simulink model "FrictionID_ref"  (R2022b)
settings: Solver=FixedStepDiscrete  StartTime=0.0  StopTime=160  FixedStep=0.000005  RelTol=1e-3  EnableMultiTasking=on
settings Model: RequirementInfo={} %GIDa_fe9045fd_0412_4b6e_8206_617cc20e6fde  FPTRunName=Active  Creator=ts  LastModifiedBy=hufnagelde
settings SolverCC: AlgebraicLoopSolver=TrustRegion  PositivePriorityOrder=on  AutoInsertRateTranBlk=on
settings DataIOCC: SaveOutput=off  SignalLogging=off  DSMLogging=off  SaveTime=off
settings OptimizationCC: DefaultParameterBehavior=Inlined  UseDivisionForNetSlopeComputation=on  GainParamInheritBuiltInType=on  UseFloatMulNetSlope=on  DefaultUnderspecifiedDataType=single  UseSpecifiedMinMax=on  InlineInvariantSignals=on  PassReuseOutputArgsAs=Individual arguments  ZeroExternalMemoryAtStartup=off  ZeroInternalMemoryAtStartup=off  NoFixptDivByZeroProtection=on  EfficientFloat2IntCast=on  LifeSpan=1  MaxStackSize=64  OptimizeBlockOrder=speed  DifferentSizesBufferReuse=on  EfficientTunableParamExpr=on
settings DebuggingCC: UnconnectedInputMsg=warning  UnconnectedOutputMsg=warning  UnconnectedLineMsg=warning  BusObjectLabelMismatch=error  AllowSymbolicDim=off  SFUnexpectedBacktrackingDiag=warning  SFNoUnconditionalDefaultTransitionDiag=warning  SFExecutionAtInitializationDiag=none  SFMachineParentedDataDiag=warning  ArithmeticOperatorsInVariantConditions=warning
settings HardwareCC: ProdBitPerPointer=32  ProdBitPerSizeT=32  ProdBitPerPtrDiffT=32  ProdLargestAtomicInteger=Long  ProdLargestAtomicFloat=Double  ProdWordSize=32  ProdLongLongMode=on  ProdHWDeviceType=ARM Compatible->ARM Cortex-R  HardwareBoardFeatureSet=SoCBlockset
settings ModelReferenceCC: EnableRefExpFcnMdlSchedulingChecks=on
settings SFSimCC: SimGenImportedTypeDefs=on  MATLABDynamicMemAlloc=off
settings RTWCC: Description=Embedded Coder  SystemTargetFile=ert.tlc  GenCodeOnly=on  TemplateMakefile=ert_default_tmf  GenerateReport=on  BuildConfiguration=Faster Runs  IncludeHyperlinkInReport=on  LaunchReport=on  GenerateTraceInfo=on  GenerateTraceReport=on  GenerateTraceReportSl=on  GenerateTraceReportSf=on  GenerateTraceReportEml=on  GenerateCodeMetricsReport=on  CheckMdlBeforeBuild=Warning  DLArmComputeVersion=19.05
settings CodeAppCC: ForceParamTrailComments=on  IgnoreCustomStorageClasses=off  OperatorAnnotations=on  SimulinkDataObjDesc=on  SFDataObjDesc=on  MATLABFcnDesc=on  CustomSymbolStrGlobalVar=rt$M$R$N  CustomSymbolStrType=$N$M$R_t  CustomSymbolStrFcn=$N$M$F  CustomSymbolStrMacro=$N$M  InsertBlockDesc=on  StateflowObjectComments=on  MATLABSourceComments=on  EnableCustomComments=on  ReqsInCode=on
settings ERTTargetCC: TargetLangStandard=C99 (ISO)  CodeReplacementLibrary=GNU C99 extensions  MultiwordLength=2048  IncludeMdlTerminateFcn=off  CombineSignalStateStructs=on  SuppressErrorStatus=on  IncludeFileDelimiter=UseQuote  SupportAbsoluteTime=off  CodeInterfacePackaging=Reusable function  SupportNonFinite=off  RemoveResetFunc=off  InlinedParameterPlacement=NonHierarchical  MultiInstanceErrorCode=Warning  RootIOFormat=Part of model data structure  ERTCustomFileTemplate=example_file_process.tlc  GlobalDataDefinition=InSourceFile  GlobalDataReference=InSourceFile  ERTFilePackagingFormat=CompactWithDataFile  SuppressUnreachableDefaultCases=off
settings ConfigComp: CovScope=ReferencedModels  CovSaveName=covdata_rollAP  CovMetricSettings=dcmtrwe  CovHTMLOptions=-sRT=1 -aTS=1 -bRG=1 -bTC=1 -hTR=1 -nFC=0 -scm=1 -bcm=1 -xEv=0  CovSaveCumulativeToWorkspaceVar=on  CovSaveSingleToWorkspaceVar=on  CovCumulativeVarName=covCumulativeData_rollAP  CovReportOnPause=off  CovExternalEMLEnable=off  CovSFcnEnable=off

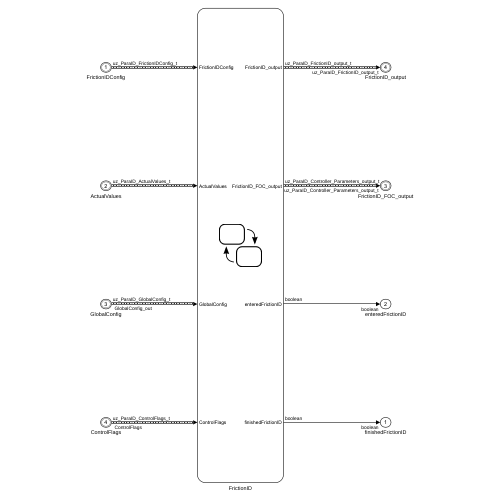
[thumbnail: Simulink's stored preview of the top-level diagram]
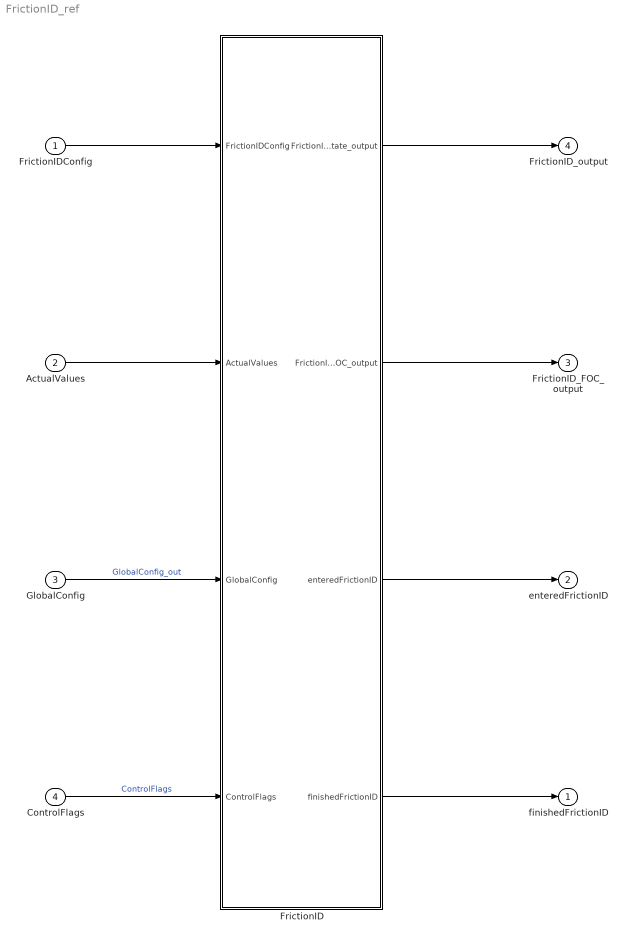
== system FrictionID_ref ==
  FrictionIDConfig : Inport  OutDataTypeStr=Bus: uz_ParaID_FrictionIDConfig_t  PortDimensions=1  SampleTime=[5.0000000000000002e-05,0]  BusOutputAsStruct=on
  ActualValues : Inport  Port=2  OutDataTypeStr=Bus: uz_ParaID_ActualValues_t  PortDimensions=1  SampleTime=[5.0000000000000002e-05,0]  BusOutputAsStruct=on
  GlobalConfig : Inport  Port=3  OutDataTypeStr=Bus: uz_ParaID_GlobalConfig_t  PortDimensions=1  SampleTime=[5.0000000000000002e-05,0]  BusOutputAsStruct=on
  ControlFlags : Inport  Port=4  OutDataTypeStr=Bus: uz_ParaID_ControlFlags_t  PortDimensions=1  SampleTime=[5.0000000000000002e-05,0]  BusOutputAsStruct=on
  FrictionID : Stateflow chart  TreatAsAtomicUnit=on
      settings: PortSchema="{\"entries\":[{\"content\":{\"sides\":[{\"content\":{\"connectorIds\":[\"In1\",\"In2\",\"In3\",\"In4\"]},\"type\":\"ConnectorPlacement.EquallySpacedRectSide\",\"uuid\":\"9228c284-4dde-45fc-9186-6f631f78e5bf\"},{\"content\":{\"connectorIds\":[\"Out4\",\"Out3\",\"Out2\",\"Out1\"],\"side\":\"RIGHT\"},\"type\":\"ConnectorPlacement.EquallySpacedRectSide\",\"uuid\":\"71961043-480b-43aa-8cdd-23d9057d5ad4\"},{\"content\":{\"connectorIds\":[],\"side\":\"TOP\"},\"type\":\"ConnectorPlacement.EquallySpacedRectSide\",\"uuid\":\"f6f3bc9d-566f-4498-bf43-24e8b901b7a7\"}]},\"type\":\"ConnectorPlacement.EquallySpacedConnector\",\"uuid\":\"83d2d7c4-30d1-4ed4-b102-cbae6a0e9817\"}],\"packageUris\":[\"http://schema.mathworks.com/mf0/Connector/R2020b\"],\"version\":\"1.0\"}"
  finishedFrictionID : Outport  OutDataTypeStr=boolean  PortDimensions=1  SampleTime=[5.0000000000000002e-05,0]
  enteredFrictionID : Outport  Port=2  OutDataTypeStr=boolean  PortDimensions=1  SampleTime=[5.0000000000000002e-05,0]
  FrictionID_FOC_output : Outport  Port=3  OutDataTypeStr=Bus: uz_ParaID_Controller_Parameters_output_t  PortDimensions=1  SampleTime=[5.0000000000000002e-05,0]  BusOutputAsStruct=on
  FrictionID_output : Outport  Port=4  OutDataTypeStr=Bus: uz_ParaID_FrictionID_output_t  PortDimensions=1  SampleTime=[5.0000000000000002e-05,0]  BusOutputAsStruct=on
  wires:
  FrictionIDConfig/1 -> FrictionID/1(FrictionIDConfig)
  ActualValues/1 -> FrictionID/2(ActualValues)
  GlobalConfig/1 -> FrictionID/3(GlobalConfig)  "GlobalConfig_out"
  ControlFlags/1 -> FrictionID/4(ControlFlags)  "ControlFlags"
  FrictionID/1(finishedFrictionID) -> finishedFrictionID/1
  FrictionID/2(enteredFrictionID) -> enteredFrictionID/1
  FrictionID/3(FrictionID_FOC_output) -> FrictionID_FOC_output/1
  FrictionID/4(FrictionID_state_output) -> FrictionID_output/1

== stateflow chart FrictionID_ref/FrictionID ==
  settings: updateMethod=DISCRETE  sampleTime=1/d_f_states
  note: Friction - identification
  state frictionID
    entry:
    initParams;
    enteredFrictionID=boolean(1);
    FrictionID_FOC_output.activeState=uint16(300);
    during:
    state ResetIntegrator1
      entry:
      counter2=uint32(1);
      FrictionID_FOC_output.activeState=uint16(320);
      during:
      FrictionID_FOC_output.resetIntegrator=boolean(1);
      counter2 = counter2 + 1;
      exit:
      FrictionID_FOC_output.enableFOC_torque=boolean(0);
      FrictionID_FOC_output.resetIntegrator=boolean(0);
    state CoulombFrictionTorqueEstimation
      entry:
      FrictionID_FOC_output.activeState = uint16(330);
      FrictionID_FOC_output.enableFOC_speed=boolean(1);
      FrictionID_FOC_output.n_ref_FOC=single(0);
      delay=single(0.1);
      meas_sum=single(zeros(3,1));
      measArray2(1:1024,1:3)=zeros(1024,3);
      omega_Brk=single(5.0);
      nextstate=uint16(0);
      counter=uint32(1);
      mean_count=single(256);
      meas_count=uint16(0);
      during:
      FrictionID_FOC_output.n_ref_FOC=n_eva;
      exit:
      line=gerade;
      FrictionID_state_output.CoulTorque=single(line(2));
      FrictionID_state_output.ViscoTorque=single(line(1));
      FrictionID_FOC_output.n_ref_FOC=single(0);
      state SmoothingCurrentAndOmega
        entry: FrictionID_FOC_output.activeState = uint16(331)
        meas_count=uint16(0);
        switcher=boolean(1);
        during:
        if(meas_count==uint32(0.02/GlobalConfig.sampleTimeISR))
        measArray2(mean_count,1)=meas_sum(1)/(0.02/GlobalConfig.sampleTimeISR);
        measArray2(mean_count,2)=meas_sum(2)/(0.02/GlobalConfig.sampleTimeISR);
        measArray2(mean_count,3)=meas_sum(3)/(0.02/GlobalConfig.sampleTimeISR);
        meas_sum=single(zeros(3,1));
        if(measArray2(mean_count,1)<((1-FrictionIDConfig.eta)*n_eva*0.1047) ||measArray2(mean_count,1)>((1+FrictionIDConfig.eta)*n_eva*0.1047))
        switcher=boolean(0);
        end
        mean_count = mean_count + 1;
        meas_count=uint16(0);
        end
        meas_count=meas_count+1;
        meas_sum(1)=meas_sum(1)+abs(ActualValues.omega_m);
        meas_sum(2)=meas_sum(2)+abs(ActualValues.i_dq.q);
        meas_sum(3)=meas_sum(3)+abs(ActualValues.i_dq.d);
      state DecreaseSpeed
        entry:
        counter2 = uint32(1);
        FrictionID_FOC_output.activeState = uint16(332)
        if(n_eva>0&&switcher==boolean(1))
        FrictionID_state_output.measArraySpeed(counter)=mean(measArray2(1:256,1));
        FrictionID_state_output.measArrayTorque(counter)=1.5*GlobalConfig.PMSM_config.polePairs*(GlobalConfig.PMSM_config.Psi_PM_Vs*mean(measArray2(1:256,2))....
        +(GlobalConfig.PMSM_config.Ld_Henry - GlobalConfig.PMSM_config.Lq_Henry)*mean(measArray2(1:256,3))*mean(measArray2(1:256,2)));
        counter=counter+1;
        n_eva=n_eva-(n_eva_step);
        elseif(n_eva>0&&switcher==boolean(0))
        switch_count = switch_count + 1;
        end
        if (n_eva>0 && switch_count>=5)
        n_eva=n_eva-(n_eva_step);
        switch_count = uint32(0);
        end
        if(abs(ActualValues.omega_m)<=omega_Brk&&counter>2)
        n_eva=single(0);
        nextstate=uint16(1);
        end
        during:
        counter2 = counter2 +1;
        exit:
        mean_count=1;
      (default) -> SmoothingCurrentAndOmega
      SmoothingCurrentAndOmega -> DecreaseSpeed : [mean_count==256]
      DecreaseSpeed -> SmoothingCurrentAndOmega : [delay_transition_counter == counter2]
    state BreakawayTorqueEstimation
      entry:
      FrictionID_FOC_output.activeState = uint16(310);
      FrictionID_FOC_output.enableFOC_torque=boolean(1);
      FrictionID_FOC_output.resetIntegrator=boolean(0);
      during:
      FrictionID_FOC_output.M_ref_FOC=M_eva;
      if(nextstate>=FrictionIDConfig.BrkCount)
      M_eva=single(0);
      if(counter<=FrictionIDConfig.N_Brk)
      Ustep(counter)=M_Brk;
      end
      nextstate=uint16(0);
      counter = counter + 1;
      end
      exit:
      FrictionID_state_output.BrkTorque=max(Ustep);
      FrictionID_FOC_output.M_ref_FOC = single(0.0);
      state waitstate
        entry:
        counter2 = uint32(1);
        FrictionID_FOC_output.activeState=uint16(311);
        during:
        counter2 = counter2 + 1;
      state increaseCurrent
        entry:
        FrictionID_FOC_output.activeState = uint16(312);
        if(abs(ActualValues.omega_m)>single(0) && M_eva>single(0))
        M_Brk=M_eva;
        nextstate=nextstate+1;
        end
        if(abs(ActualValues.omega_m)<=omega_Brk&&abs(M_eva)<FrictionIDConfig.maxCurrent)
        M_eva=M_eva+M_eva_step;
        nextstate=uint16(0);
        end
      (default) -> waitstate
      increaseCurrent -> waitstate
      waitstate -> increaseCurrent : [delay_transition_counter == counter2]
    state FinishDataTransfer
      entry:
      counter2=uint32(1);
      FrictionID_FOC_output.resetIntegrator=boolean(1);
      FrictionID_FOC_output.activeState=uint16(341);
      during:
      counter2 = counter2 +1;
      exit:
      finishedFrictionID=boolean(1);
      enteredFrictionID=boolean(0);
      reset_FOC_output;
    state ResetIntegrator
      entry:
      counter2=uint32(1);
      FrictionID_FOC_output.activeState=uint16(340);
      during:
      counter2 = counter2 +1;
      FrictionID_FOC_output.resetIntegrator=boolean(1);
      exit:
    BreakawayTorqueEstimation -> ResetIntegrator1 : [counter>FrictionIDConfig.N_Brk]
    ResetIntegrator1 -> CoulombFrictionTorqueEstimation : [one_sec_transition_counter == counter2]
    (default) -> BreakawayTorqueEstimation
    CoulombFrictionTorqueEstimation -> ResetIntegrator : [nextstate==1]
    ResetIntegrator -> FinishDataTransfer : [ten_sec_transition_counter == counter2]
  state Waiting
    entry:
    %wait for activation of
    %FrictionID
    %donothing
  note: ---
  Waiting -> frictionID [order 1] : [ControlFlags.startFrictionID==1 && GlobalConfig.Reset==0 && GlobalConfig.ACCEPT==1]
  (default) -> Waiting
  Waiting -> Waiting [order 2] : [GlobalConfig.Reset==1]{finishedFrictionID=boolean(0);
      | enteredFrictionID=boolean(0);
      | initParams;}
  frictionID -> Waiting : [GlobalConfig.Reset==1 || GlobalConfig.FrictionID==0 || ....
      | GlobalConfig.enableParameterID==0]
      | {enteredFrictionID=boolean(0);initParams;}
  FinishDataTransfer -> Waiting : [one_sec_transition_counter == counter2]
  data: u function_output single size=[2 1]; counter local; measArray2 local; Ustep local; delay local; M_Brk local; M_eva local; M_eva_step local; line local single size=[2 1]; mean_count local single; meas_count local; meas_sum local; nextstate local; omega_Brk local; switcher local boolean; finishedFrictionID output boolean; enteredFrictionID output boolean; FrictionIDConfig input Bus: uz_ParaID_FrictionIDConfig_t; FrictionID_FOC_output output Bus: uz_ParaID_Controller_Parameters_output_t; ActualValues input Bus: uz_ParaID_ActualValues_t; GlobalConfig input Bus: uz_ParaID_GlobalConfig_t; ControlFlags input Bus: uz_ParaID_ControlFlags_t; FrictionID_state_output output Bus: uz_ParaID_FrictionID_output_t; n_eva_step local; n_eva local; one_sec_transition_counter local; delay_transition_counter local; counter2 local; ten_sec_transition_counter local; switch_count local
  function u=gerade:
    | function u=gerade
    | 
    | %Evaluation of Coulomb and viscous torque 
    | %using a linear regression line
    | 
    | %--------initalizing---------------------------------------
    | gerade=single(zeros(2,1));
    | zaehler=single(0);
    | measSum=single(0);
    | iestSum=single(0);
    | Xy=single(0);
    | Xx=single(0);
    | meanMeas=single(0);
    | meanIest=single(0);
    | SS_xy=single(0);
    | SS_xx=single(0);
    | 
    | %--------summing up----------------------------------
    | for k=single(2):single(255)
    |     
    |     %----------reject outliers---------------------------
    |     if (FrictionID_state_output.measArraySpeed(k) >5 && ( FrictionID_state_output.measArrayTorque(k)<1.3*FrictionID_state_output.measArrayTorque(k+1)....
    |             || FrictionID_state_output.measArrayTorque(k)<1.3*FrictionID_state_output.measArrayTorque(k-1) ) &&....
    |             ( FrictionID_state_output.measArrayTorque(k)>FrictionID_state_output.measArrayTorque(k+1)*0.7  ||....
    |             FrictionID_state_output.measArrayTorque(k)>FrictionID_state_output.measArrayTorque(k-1)*0.7 )  )
    |         zaehler=zaehler+1;
    |         measSum=measSum+FrictionID_state_output.measArraySpeed(k);
    |         iestSum=iestSum+FrictionID_state_output.measArrayTorque(k);        
    |         Xy=FrictionID_state_output.measArraySpeed(k)*FrictionID_state_output.measArrayTorque(k)+Xy;
    |         Xx=FrictionID_state_output.measArraySpeed(k)*FrictionID_state_output.measArraySpeed(k)+Xx;
    |     end
    |        
    | end
    | 
    | %-------calculate mean-------------------------------
    | meanMeas=measSum/zaehler;
    | meanIest=iestSum/zaehler;
    | 
    | %----------calculate varianz--------------------------
    |     SS_xy = Xy-zaehler*meanMeas*meanIest; 
    |     SS_xx = Xx- zaehler*meanMeas*meanMeas; 
    | 
    | %-------viscous friction-------------------------------    
    | gerade(1)=single(SS_xy/SS_xx);
    | 
    | %-------Coulomb friction-----------------------------
    | gerade(2)=single(meanIest-(SS_xy/SS_xx)*meanMeas);
    | 
    | u=gerade;
    | end
  function initParams:
    | function initParams
    | 
    | %This is used instead of "after(1.0,sec) to ensure the same transition time
    | %independelty of the sampletime in the c-code
    | one_sec_transition_counter = uint32(1/GlobalConfig.sampleTimeISR);
    | ten_sec_transition_counter = uint32(10/GlobalConfig.sampleTimeISR);
    | delay_transition_counter = uint32(single(5*(GlobalConfig.Kp_iq / GlobalConfig.Ki_iq))/GlobalConfig.sampleTimeISR);
    | % initialize variables
    | meas_sum            = single(zeros(3,1));
    | measArray2 			= single(zeros(2048,3));
    | counter             = uint32(1);
    | switch_count        = uint32(0);
    | Ustep               = single(zeros(103,1));
    | nextstate           = uint16(0);
    | M_eva               = single(0);
    | n_eva               = single(FrictionIDConfig.n_eva_max);
    | n_eva_step          = single(n_eva/single(FrictionIDConfig.N_Visco));
    | M_Brk               = single(0);
    | mean_count          = single(0);
    | omega_Brk           = single(1);
    | delay               = single(5*(GlobalConfig.Kp_iq / GlobalConfig.Ki_iq));
    | M_eva_step          = single(GlobalConfig.ratTorque*FrictionIDConfig.StepScale);
    | line                = single(zeros(2,1));
    | 
    | %Outputs
    | FrictionID_FOC_output.n_ref_FOC             = single(0.0);
    | FrictionID_FOC_output.M_ref_FOC             = single(0.0);
    | FrictionID_FOC_output.i_dq_ref.d            = single(0.0);
    | FrictionID_FOC_output.i_dq_ref.q            = single(M_eva);
    | FrictionID_FOC_output.i_dq_ref.zero         = single(0.0);
    | FrictionID_FOC_output.enableFOC_speed       = boolean(0);
    | FrictionID_FOC_output.enableFOC_current     = boolean(0);
    | FrictionID_FOC_output.enableFOC_torque      = boolean(0);
    | FrictionID_FOC_output.resetIntegrator       = boolean(1);
    | finishedFrictionID                          = boolean(0);
    | FrictionID_FOC_output.Kp_id_out             = single(GlobalConfig.Kp_id);
    | FrictionID_FOC_output.Kp_iq_out             = single(GlobalConfig.Kp_iq);
    | FrictionID_FOC_output.Kp_n_out              = single(GlobalConfig.Kp_n);
    | FrictionID_FOC_output.Ki_id_out             = single(GlobalConfig.Ki_id);
    | FrictionID_FOC_output.Ki_iq_out             = single(GlobalConfig.Ki_iq);
    | FrictionID_FOC_output.Ki_n_out              = single(GlobalConfig.Ki_n);
    | FrictionID_FOC_output.activeState           = uint16(0);
    | 
    | FrictionID_state_output.BrkTorque                 = single(0.0);
    | FrictionID_state_output.CoulTorque                = single(0.0);
    | FrictionID_state_output.ViscoTorque               = single(0.0);
    | FrictionID_state_output.measArraySpeed			= single(zeros(256,1));
    | FrictionID_state_output.measArrayTorque           = single(zeros(256,1));
    | end
  function reset_FOC_output:
    | function reset_FOC_output
    | 
    | %Outputs
    | FrictionID_FOC_output.n_ref_FOC             = single(0.0);
    | FrictionID_FOC_output.M_ref_FOC             = single(0.0);
    | FrictionID_FOC_output.i_dq_ref.d            = single(0.0);
    | FrictionID_FOC_output.i_dq_ref.q            = single(M_eva);
    | FrictionID_FOC_output.i_dq_ref.zero         = single(0.0);
    | FrictionID_FOC_output.enableFOC_speed       = boolean(0);
    | FrictionID_FOC_output.enableFOC_current     = boolean(0);
    | FrictionID_FOC_output.enableFOC_torque      = boolean(0);
    | FrictionID_FOC_output.resetIntegrator       = boolean(1);
    | FrictionID_FOC_output.Kp_id_out             = single(GlobalConfig.Kp_id);
    | FrictionID_FOC_output.Kp_iq_out             = single(GlobalConfig.Kp_iq);
    | FrictionID_FOC_output.Kp_n_out              = single(GlobalConfig.Kp_n);
    | FrictionID_FOC_output.Ki_id_out             = single(GlobalConfig.Ki_id);
    | FrictionID_FOC_output.Ki_iq_out             = single(GlobalConfig.Ki_iq);
    | FrictionID_FOC_output.Ki_n_out              = single(GlobalConfig.Ki_n);
    | FrictionID_FOC_output.activeState               = uint16(0);
    | end
